simulink model "model_sim_CHBjt7"  (R2023b)
settings: Solver=ode3  StartTime=0.0  StopTime=5  FixedStep=01e-6  RelTol=1e-3
InitFcn:
  | sysinit
StopFcn:
  | code_CHBJT7_stopfcn
values from neighbouring files (symbols this model uses):
  C = 0.0234    [sysinit.m]
  f = 50    [sysinit.m]
  f_switch = 250    [sysinit.m]
  fn = 50    [sysinit.m]
  L = 0.002    [sysinit.m]
  L_1 = eps    [simout_chb_par.m]    (also in simout_chbjt_par.m; sysinit.m)
  L_ori = 0.02    [sysinit.m]
  L_sec = 0.06    [sysinit.m]
  m = 0.95    [sysinit.m]
  P0 = 8e6    (= 8000000)    [sysinit.m]
  R = 1.5    [sysinit.m]
  Source_Amp = 10000    [sysinit.m]
  st = 1e-6    (= 1e-06)    [sysinit.m]
  Td = 15e-7    (= 1.5e-06)    [sysinit.m]
  Ts2 = 0.5e-3    (= 0.0005)    [sysinit.m]
  U_dcN = 2500    [sysinit.m]
  Ul_in = 1900    [sysinit.m]
undefined symbols (not defined in the file or in its folder): magnitude
libraries: spsSeriesRLCBranchLib x120, spsDiodeLib x45, spsIGBTLib x36, spsMeanLib x20, spsCurrentMeasurementLib x15, spsThreePhaseVIMeasurementLib x10, spsOnDelayLib x9, spsMultiWindingTransformerLib x9, spsUniversalBridgeLib x9, simulink x5, spsVoltageMeasurementLib x5, spsRMSLib x4
(part 3 of 3)

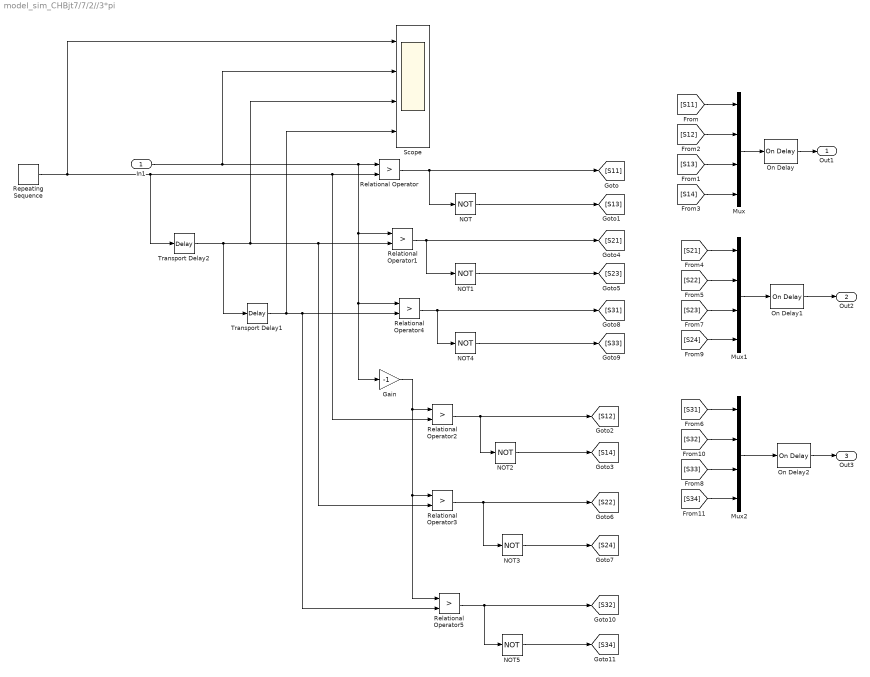
== system model_sim_CHBjt7/7/2//3*pi ==
  In1 : Inport
  Gain : Gain  Gain=-1
  Mux : Mux
  Mux1 : Mux
  Mux2 : Mux
  NOT{,1..5} (6 alike) : Logic  Operator=NOT  AllPortsSameDT=off  OutDataTypeStr=boolean
  On Delay : spsOnDelayLib/On Delay  DelayType=On delay  delay=ttd  ic=0  Ts=0
  On Delay1 : spsOnDelayLib/On Delay  DelayType=On delay  delay=ttd  ic=0  Ts=0
  On Delay2 : spsOnDelayLib/On Delay  DelayType=On delay  delay=ttd  ic=0  Ts=0
  Relational Operator{,1..5} (6 alike) : RelationalOperator  Operator=>  OutDataTypeStr=boolean  RndMeth=Simplest  InputSameDT=off
  Repeating Sequence : simulink/Sources/Repeating Sequence  rep_seq_t=[0 0.5 1]/f_car  rep_seq_y=[-1 1 -1]*1000
  Scope : Scope  NumInputPorts=4
  Transport Delay1 : TransportDelay  DelayTime=tt/f_car  BufferSize=3072
  Transport Delay2 : TransportDelay  DelayTime=tt/f_car  BufferSize=3072
  Out1 : Outport
  Out2 : Outport  Port=2
  Out3 : Outport  Port=3
  wires:
  NOT/1 -> [S13]
  Transport Delay2/1 -> Scope/3, Relational Operator3/2, Relational Operator1/2, Transport Delay1/1
  [S14] -> Mux/4
  [S23] -> Mux1/3
  [S12] -> Mux/2
  In1/1 -> Scope/2, Relational Operator4/1, Gain/1, Relational Operator1/1, Relational Operator/1
  [S34] -> Mux2/4
  [S32] -> Mux2/2
  Mux2/1 -> On Delay2/1
  Relational Operator5/1 -> [S32], NOT5/1
  NOT2/1 -> [S14]
  [S21] -> Mux1/1
  NOT4/1 -> [S33]
  Relational Operator1/1 -> NOT1/1, [S21]
  [S22] -> Mux1/2
  [S33] -> Mux2/3
  NOT3/1 -> [S24]
  Mux/1 -> On Delay/1
  [S24] -> Mux1/4
  Relational Operator4/1 -> [S31], NOT4/1
  Gain/1 -> Relational Operator5/1, Relational Operator3/1, Relational Operator2/1
  [S13] -> Mux/3
  Relational Operator2/1 -> NOT2/1, [S12]
  [S31] -> Mux2/1
  [S11] -> Mux/1
  NOT5/1 -> [S34]
  Relational Operator/1 -> NOT/1, [S11]
  NOT1/1 -> [S23]
  Mux1/1 -> On Delay1/1
  Relational Operator3/1 -> NOT3/1, [S22]
  On Delay/1 -> Out1/1
  On Delay1/1 -> Out2/1
  On Delay2/1 -> Out3/1
  Transport Delay1/1 -> Scope/4, Relational Operator5/2, Relational Operator4/2
  Repeating Sequence/1 -> Scope/1, Transport Delay2/1, Relational Operator2/2, Relational Operator/2

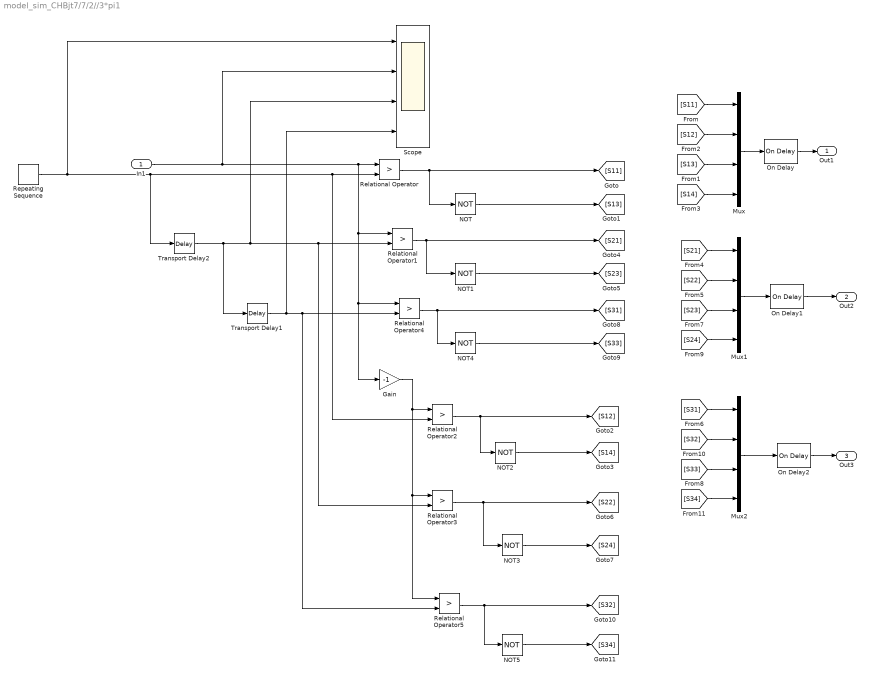
== system model_sim_CHBjt7/7/2//3*pi1 ==
  In1 : Inport
  Gain : Gain  Gain=-1
  Mux : Mux
  Mux1 : Mux
  Mux2 : Mux
  NOT{,1..5} (6 alike) : Logic  Operator=NOT  AllPortsSameDT=off  OutDataTypeStr=boolean
  On Delay : spsOnDelayLib/On Delay  DelayType=On delay  delay=ttd  ic=0  Ts=0
  On Delay1 : spsOnDelayLib/On Delay  DelayType=On delay  delay=ttd  ic=0  Ts=0
  On Delay2 : spsOnDelayLib/On Delay  DelayType=On delay  delay=ttd  ic=0  Ts=0
  Relational Operator{,1..5} (6 alike) : RelationalOperator  Operator=>  OutDataTypeStr=boolean  RndMeth=Simplest  InputSameDT=off
  Repeating Sequence : simulink/Sources/Repeating Sequence  rep_seq_t=[0 0.5 1]/f_car  rep_seq_y=[-1 1 -1]*1000
  Scope : Scope  NumInputPorts=4
  Transport Delay1 : TransportDelay  DelayTime=tt/f_car  BufferSize=3072
  Transport Delay2 : TransportDelay  DelayTime=tt/f_car  BufferSize=3072
  Out1 : Outport
  Out2 : Outport  Port=2
  Out3 : Outport  Port=3
  wires:
  NOT/1 -> [S13]
  Transport Delay2/1 -> Scope/3, Relational Operator3/2, Relational Operator1/2, Transport Delay1/1
  [S14] -> Mux/4
  [S23] -> Mux1/3
  [S12] -> Mux/2
  In1/1 -> Scope/2, Relational Operator4/1, Gain/1, Relational Operator1/1, Relational Operator/1
  [S34] -> Mux2/4
  [S32] -> Mux2/2
  Mux2/1 -> On Delay2/1
  Relational Operator5/1 -> [S32], NOT5/1
  NOT2/1 -> [S14]
  [S21] -> Mux1/1
  NOT4/1 -> [S33]
  Relational Operator1/1 -> NOT1/1, [S21]
  [S22] -> Mux1/2
  [S33] -> Mux2/3
  NOT3/1 -> [S24]
  Mux/1 -> On Delay/1
  [S24] -> Mux1/4
  Relational Operator4/1 -> [S31], NOT4/1
  Gain/1 -> Relational Operator5/1, Relational Operator3/1, Relational Operator2/1
  [S13] -> Mux/3
  Relational Operator2/1 -> NOT2/1, [S12]
  [S31] -> Mux2/1
  [S11] -> Mux/1
  NOT5/1 -> [S34]
  Relational Operator/1 -> NOT/1, [S11]
  NOT1/1 -> [S23]
  Mux1/1 -> On Delay1/1
  Relational Operator3/1 -> NOT3/1, [S22]
  On Delay/1 -> Out1/1
  On Delay1/1 -> Out2/1
  On Delay2/1 -> Out3/1
  Transport Delay1/1 -> Scope/4, Relational Operator5/2, Relational Operator4/2
  Repeating Sequence/1 -> Scope/1, Transport Delay2/1, Relational Operator2/2, Relational Operator/2

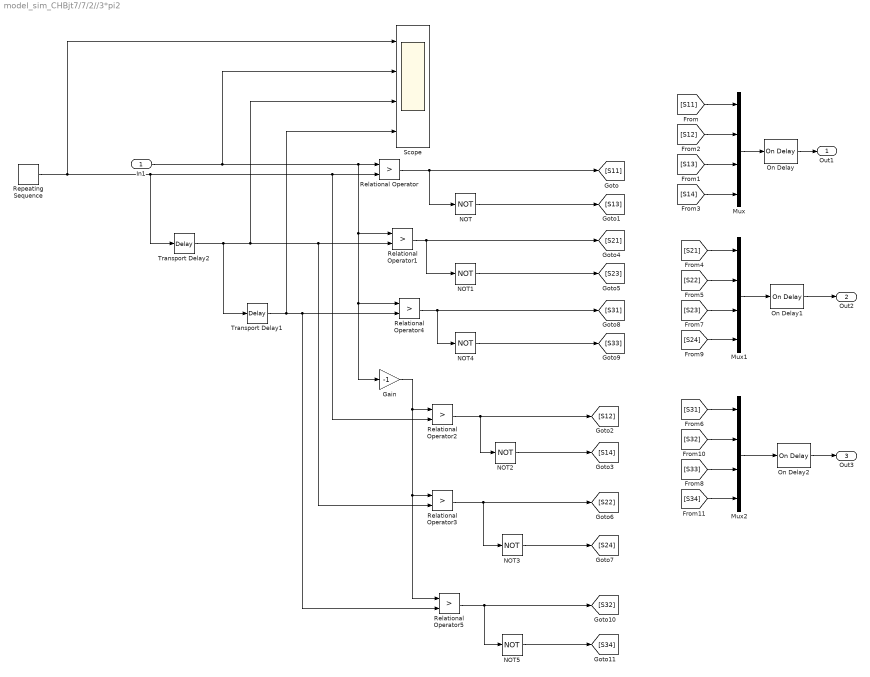
== system model_sim_CHBjt7/7/2//3*pi2 ==
  In1 : Inport
  Gain : Gain  Gain=-1
  Mux : Mux
  Mux1 : Mux
  Mux2 : Mux
  NOT{,1..5} (6 alike) : Logic  Operator=NOT  AllPortsSameDT=off  OutDataTypeStr=boolean
  On Delay : spsOnDelayLib/On Delay  DelayType=On delay  delay=ttd  ic=0  Ts=0
  On Delay1 : spsOnDelayLib/On Delay  DelayType=On delay  delay=ttd  ic=0  Ts=0
  On Delay2 : spsOnDelayLib/On Delay  DelayType=On delay  delay=ttd  ic=0  Ts=0
  Relational Operator{,1..5} (6 alike) : RelationalOperator  Operator=>  OutDataTypeStr=boolean  RndMeth=Simplest  InputSameDT=off
  Repeating Sequence : simulink/Sources/Repeating Sequence  rep_seq_t=[0 0.5 1]/f_car  rep_seq_y=[-1 1 -1]*1000
  Scope : Scope  NumInputPorts=4
  Transport Delay1 : TransportDelay  DelayTime=tt/f_car  BufferSize=3072
  Transport Delay2 : TransportDelay  DelayTime=tt/f_car  BufferSize=3072
  Out1 : Outport
  Out2 : Outport  Port=2
  Out3 : Outport  Port=3
  wires:
  NOT/1 -> [S13]
  Transport Delay2/1 -> Scope/3, Relational Operator3/2, Relational Operator1/2, Transport Delay1/1
  [S14] -> Mux/4
  [S23] -> Mux1/3
  [S12] -> Mux/2
  In1/1 -> Scope/2, Relational Operator4/1, Gain/1, Relational Operator1/1, Relational Operator/1
  [S34] -> Mux2/4
  [S32] -> Mux2/2
  Mux2/1 -> On Delay2/1
  Relational Operator5/1 -> [S32], NOT5/1
  NOT2/1 -> [S14]
  [S21] -> Mux1/1
  NOT4/1 -> [S33]
  Relational Operator1/1 -> NOT1/1, [S21]
  [S22] -> Mux1/2
  [S33] -> Mux2/3
  NOT3/1 -> [S24]
  Mux/1 -> On Delay/1
  [S24] -> Mux1/4
  Relational Operator4/1 -> [S31], NOT4/1
  Gain/1 -> Relational Operator5/1, Relational Operator3/1, Relational Operator2/1
  [S13] -> Mux/3
  Relational Operator2/1 -> NOT2/1, [S12]
  [S31] -> Mux2/1
  [S11] -> Mux/1
  NOT5/1 -> [S34]
  Relational Operator/1 -> NOT/1, [S11]
  NOT1/1 -> [S23]
  Mux1/1 -> On Delay1/1
  Relational Operator3/1 -> NOT3/1, [S22]
  On Delay/1 -> Out1/1
  On Delay1/1 -> Out2/1
  On Delay2/1 -> Out3/1
  Transport Delay1/1 -> Scope/4, Relational Operator5/2, Relational Operator4/2
  Repeating Sequence/1 -> Scope/1, Transport Delay2/1, Relational Operator2/2, Relational Operator/2

== system model_sim_CHBjt7/7/Subsystem ==
  In1 : Inport
  In2 : Inport  Port=2
  In3 : Inport  Port=3
  Add{1..3,9} (4 alike) : Sum
  Gain : Gain  Gain=-0.5
  Max : MinMax  Function=max  Inputs=3
  Max1 : MinMax  Inputs=3
  Out1 : Outport
  Out2 : Outport  Port=2
  Out3 : Outport  Port=3
  wires:
  In2/1 -> Add3/2, Max1/2, Max/2
  In3/1 -> Add9/2, Max1/3, Max/3
  In1/1 -> Max1/1, Add2/2, Max/1
  Gain/1 -> Add9/1, Add3/1, Add2/1
  Max/1 -> Add1/1
  Max1/1 -> Add1/2
  Add1/1 -> Gain/1
  Add9/1 -> Out3/1
  Add2/1 -> Out1/1
  Add3/1 -> Out2/1

== system model_sim_CHBjt7/JUNCTION TEMP/Subsystem14 ==
  In1 : Inport
  In2 : Inport  Port=2
  Add : Sum
  Constant : Constant  Value=0
  Constant1 : Constant  Value=0
  Gain1 : Gain  Gain=0.39e-3
  Gain2 : Gain  Gain=1.39
  Gain3 : Gain
  Logical Operator : Logic  AllPortsSameDT=off  OutDataTypeStr=boolean
  Math Function : Math  Operator=magnitude^2  SignedPower=on
  Relational Operator : RelationalOperator  Operator=>  OutDataTypeStr=boolean  RndMeth=Simplest  InputSameDT=off
  Switch13 : Switch  Criteria=u2 > Threshold  SaturateOnIntegerOverflow=off  InputSameDT=off
  t1_temper{1..4} (4 alike) : Scope
  Out1 : Outport  VectorParamsAs1DForOutWhenUnconnected=off
  wires:
  Add/1 -> t1_temper4/1, Switch13/1
  Gain2/1 -> Add/2
  Math Function/1 -> Gain1/1
  In1/1 -> t1_temper3/1, Relational Operator/1, Gain3/1
  Gain1/1 -> Add/1
  Gain3/1 -> Gain2/1, Math Function/1
  Constant/1 -> Relational Operator/2
  Relational Operator/1 -> Logical Operator/1
  In2/1 -> t1_temper1/1, Logical Operator/2
  Logical Operator/1 -> t1_temper2/1, Switch13/2
  Switch13/1 -> Out1/1
  Constant1/1 -> Switch13/3

== system model_sim_CHBjt7/JUNCTION TEMP/Subsystem15 ==
  In1 : Inport
  In2 : Inport  Port=2
  Add1 : Sum  Inputs=5
  Add2 : Sum  Inputs=+++
  Add3 : Sum
  Constant1 : Constant  Value=40
  Discrete Filter1 : DiscreteFilter  Numerator=[Ts2/0.3]  Denominator=[1 (Ts2/0.3)-1]  SampleTime=Ts2
  Discrete Filter5 : DiscreteFilter  Numerator=[Ts2/605e-3]  Denominator=[1 (Ts2/605e-3)-1]  SampleTime=Ts2
  Discrete Filter6 : DiscreteFilter  Numerator=[Ts2/101e-3]  Denominator=[1 (Ts2/101e-3)-1]  SampleTime=Ts2
  Discrete Filter7 : DiscreteFilter  Numerator=[Ts2/5.2e-3]  Denominator=[1 (Ts2/5.2e-3)-1]  SampleTime=Ts2
  Discrete Filter8 : DiscreteFilter  Numerator=[Ts2/0.6e-3]  Denominator=[1 (Ts2/0.6e-3)-1]  SampleTime=Ts2
  Discrete Filter9 : DiscreteFilter  Numerator=[Ts2/0.5]  Denominator=[1 (Ts2/0.5)-1]  SampleTime=Ts2
  Gain1 : Gain  Gain=2.4e-3
  Gain5 : Gain  Gain=3.45e-3
  Gain6 : Gain  Gain=2.26e-3
  Gain7 : Gain  Gain=0.97e-3
  Gain8 : Gain  Gain=0.1e-3
  Gain9 : Gain  Gain=7.5e-3
  Out1 : Outport  VectorParamsAs1DForOutWhenUnconnected=off
  wires:
  In1/1 -> Add3/1
  In2/1 -> Add3/2
  Gain6/1 -> Discrete Filter6/1
  Gain9/1 -> Discrete Filter9/1
  Discrete Filter9/1 -> Add2/1
  Gain5/1 -> Discrete Filter5/1
  Discrete Filter6/1 -> Add1/2
  Gain7/1 -> Discrete Filter7/1
  Constant1/1 -> Add2/3
  Discrete Filter7/1 -> Add1/3
  Discrete Filter8/1 -> Add1/4
  Discrete Filter5/1 -> Add1/1
  Gain8/1 -> Discrete Filter8/1
  Add1/1 -> Add2/2
  Add2/1 -> Out1/1
  Discrete Filter1/1 -> Add1/5
  Gain1/1 -> Discrete Filter1/1
  Add3/1 -> Gain5/1, Gain9/1, Gain6/1, Gain7/1, Gain1/1, Gain8/1

== system model_sim_CHBjt7/JUNCTION TEMP/Subsystem16 ==
  In1 : Inport
  In2 : Inport  Port=2
  Abs1 : Abs  SaturateOnIntegerOverflow=off
  Add : Sum
  Constant1 : Constant  Value=0
  Constant2 : Constant  Value=0
  Gain1 : Gain  Gain=21.5/4000*U_dcN/2800
  Gain2 : Gain  Gain=3/4000*U_dcN/2800
  Gain3 : Gain  Gain=1/Ts2
  Gain4 : Gain
  Logical Operator : Logic  AllPortsSameDT=off  OutDataTypeStr=boolean
  Logical Operator1 : Logic  Operator=NOT  AllPortsSameDT=off  OutDataTypeStr=boolean
  Logical Operator2 : Logic  Operator=NOT  AllPortsSameDT=off  OutDataTypeStr=boolean
  Logical Operator3 : Logic  AllPortsSameDT=off  OutDataTypeStr=boolean
  Logical Operator4 : Logic  AllPortsSameDT=off  OutDataTypeStr=boolean
  Logical Operator5 : Logic  Operator=NOT  AllPortsSameDT=off  OutDataTypeStr=boolean
  Pulse Generator : DiscretePulseGenerator  PulseType=Time based  Period=Ts2  PulseWidth=5
  Scope1 : Scope  NumInputPorts=3
  Scope7 : Scope  NumInputPorts=2
  Switch{1..4} (4 alike) : Switch  Criteria=u2 > Threshold  SaturateOnIntegerOverflow=off  InputSameDT=off
  Unit Delay{,1..3} (4 alike) : UnitDelay  SampleTime=1e-6  HasFrameUpgradeWarning=on
  Out1 : Outport  VectorParamsAs1DForOutWhenUnconnected=off
  wires:
  In2/1 -> Logical Operator2/1, Logical Operator/1, Unit Delay/1
  Logical Operator/1 -> Switch1/2
  Abs1/1 -> Add/1
  Switch2/1 -> Gain1/1
  Switch1/1 -> Scope1/1, Abs1/1
  Unit Delay/1 -> Logical Operator3/1, Logical Operator1/1
  Logical Operator1/1 -> Logical Operator/2
  Logical Operator2/1 -> Logical Operator3/2
  Logical Operator3/1 -> Switch2/2
  Constant2/1 -> Switch2/3
  Gain2/1 -> Switch1/1
  Gain1/1 -> Switch1/3
  Switch3/1 -> Add/2
  Constant1/1 -> Switch3/1
  Pulse Generator/1 -> Unit Delay3/1, Logical Operator4/1
  Switch4/1 -> Scope7/2, Unit Delay2/1, Gain3/1
  Unit Delay2/1 -> Switch4/3
  Unit Delay3/1 -> Logical Operator5/1
  Logical Operator5/1 -> Logical Operator4/2
  Logical Operator4/1 -> Scope1/3, Switch4/2, Switch3/2
  Unit Delay1/1 -> Scope7/1, Switch3/3, Switch4/1
  Gain3/1 -> Out1/1
  In1/1 -> Gain4/1
  Add/1 -> Scope1/2, Unit Delay1/1
  Gain4/1 -> Switch2/1, Gain2/1

== system model_sim_CHBjt7/JUNCTION TEMP/Subsystem17 ==
  In1 : Inport
  In2 : Inport  Port=2
  Add : Sum
  Constant : Constant  Value=0
  Constant1 : Constant  Value=0
  Gain1 : Gain  Gain=0.39e-3
  Gain2 : Gain  Gain=1.39
  Gain3 : Gain
  Logical Operator : Logic  AllPortsSameDT=off  OutDataTypeStr=boolean
  Math Function : Math  Operator=magnitude^2  SignedPower=on
  Relational Operator : RelationalOperator  Operator=>  OutDataTypeStr=boolean  RndMeth=Simplest  InputSameDT=off
  Switch13 : Switch  Criteria=u2 > Threshold  SaturateOnIntegerOverflow=off  InputSameDT=off
  t1_temper{1..4} (4 alike) : Scope
  Out1 : Outport  VectorParamsAs1DForOutWhenUnconnected=off
  wires:
  Add/1 -> t1_temper4/1, Switch13/1
  Gain2/1 -> Add/2
  Math Function/1 -> Gain1/1
  In1/1 -> t1_temper3/1, Relational Operator/1, Gain3/1
  Gain1/1 -> Add/1
  Gain3/1 -> Gain2/1, Math Function/1
  Constant/1 -> Relational Operator/2
  Relational Operator/1 -> Logical Operator/1
  In2/1 -> t1_temper1/1, Logical Operator/2
  Logical Operator/1 -> t1_temper2/1, Switch13/2
  Switch13/1 -> Out1/1
  Constant1/1 -> Switch13/3

== system model_sim_CHBjt7/JUNCTION TEMP/Subsystem18 ==
  In1 : Inport
  In2 : Inport  Port=2
  Add1 : Sum  Inputs=5
  Add2 : Sum  Inputs=+++
  Add3 : Sum
  Constant1 : Constant  Value=40
  Discrete Filter1 : DiscreteFilter  Numerator=[Ts2/0.3]  Denominator=[1 (Ts2/0.3)-1]  SampleTime=Ts2
  Discrete Filter5 : DiscreteFilter  Numerator=[Ts2/605e-3]  Denominator=[1 (Ts2/605e-3)-1]  SampleTime=Ts2
  Discrete Filter6 : DiscreteFilter  Numerator=[Ts2/101e-3]  Denominator=[1 (Ts2/101e-3)-1]  SampleTime=Ts2
  Discrete Filter7 : DiscreteFilter  Numerator=[Ts2/5.2e-3]  Denominator=[1 (Ts2/5.2e-3)-1]  SampleTime=Ts2
  Discrete Filter8 : DiscreteFilter  Numerator=[Ts2/0.6e-3]  Denominator=[1 (Ts2/0.6e-3)-1]  SampleTime=Ts2
  Discrete Filter9 : DiscreteFilter  Numerator=[Ts2/0.5]  Denominator=[1 (Ts2/0.5)-1]  SampleTime=Ts2
  Gain1 : Gain  Gain=2.4e-3
  Gain5 : Gain  Gain=3.45e-3
  Gain6 : Gain  Gain=2.26e-3
  Gain7 : Gain  Gain=0.97e-3
  Gain8 : Gain  Gain=0.1e-3
  Gain9 : Gain  Gain=7.5e-3
  Out1 : Outport  VectorParamsAs1DForOutWhenUnconnected=off
  wires:
  In1/1 -> Add3/1
  In2/1 -> Add3/2
  Gain6/1 -> Discrete Filter6/1
  Gain9/1 -> Discrete Filter9/1
  Discrete Filter9/1 -> Add2/1
  Gain5/1 -> Discrete Filter5/1
  Discrete Filter6/1 -> Add1/2
  Gain7/1 -> Discrete Filter7/1
  Constant1/1 -> Add2/3
  Discrete Filter7/1 -> Add1/3
  Discrete Filter8/1 -> Add1/4
  Discrete Filter5/1 -> Add1/1
  Gain8/1 -> Discrete Filter8/1
  Add1/1 -> Add2/2
  Add2/1 -> Out1/1
  Discrete Filter1/1 -> Add1/5
  Gain1/1 -> Discrete Filter1/1
  Add3/1 -> Gain5/1, Gain9/1, Gain6/1, Gain7/1, Gain1/1, Gain8/1

== system model_sim_CHBjt7/JUNCTION TEMP/Subsystem48 ==
  In1 : Inport
  In2 : Inport  Port=2
  Abs1 : Abs  SaturateOnIntegerOverflow=off
  Add : Sum
  Constant1 : Constant  Value=0
  Constant2 : Constant  Value=0
  Fcn2 : Fcn  Expr=-2.8E-7*u*u+0.00278*u+3.056
  Gain1 : Gain  Gain=U_dcN/2800*11.5/13
  Gain2 : Gain  Gain=4.1/500
  Gain3 : Gain  Gain=1/Ts2
  Gain4 : Gain
  Logical Operator2 : Logic  Operator=NOT  AllPortsSameDT=off  OutDataTypeStr=boolean
  Logical Operator3 : Logic  AllPortsSameDT=off  OutDataTypeStr=boolean
  Logical Operator4 : Logic  AllPortsSameDT=off  OutDataTypeStr=boolean
  Logical Operator5 : Logic  Operator=NOT  AllPortsSameDT=off  OutDataTypeStr=boolean
  Pulse Generator : DiscretePulseGenerator  PulseType=Time based  Period=Ts2  PulseWidth=5
  Saturation : Saturate  UpperLimit=5500  LowerLimit=0
  Saturation1 : Saturate  UpperLimit=100  LowerLimit=0
  Scope1 : Scope  NumInputPorts=3
  Scope7 : Scope  NumInputPorts=2
  Switch1 : Switch  Criteria=u2 > Threshold  Threshold=500  SaturateOnIntegerOverflow=off  InputSameDT=off
  Switch2 : Switch  Criteria=u2 > Threshold  SaturateOnIntegerOverflow=off  InputSameDT=off
  Switch3 : Switch  Criteria=u2 > Threshold  SaturateOnIntegerOverflow=off  InputSameDT=off
  Switch4 : Switch  Criteria=u2 > Threshold  SaturateOnIntegerOverflow=off  InputSameDT=off
  Unit Delay{,1..3} (4 alike) : UnitDelay  SampleTime=1e-6  HasFrameUpgradeWarning=on
  Out1 : Outport  VectorParamsAs1DForOutWhenUnconnected=off
  wires:
  Abs1/1 -> Add/1
  Switch2/1 -> Gain1/1
  Gain1/1 -> Abs1/1, Scope1/1
  In2/1 -> Logical Operator3/1, Unit Delay/1
  Logical Operator2/1 -> Logical Operator3/2
  Logical Operator3/1 -> Switch2/2
  Constant2/1 -> Switch2/3
  Switch3/1 -> Add/2
  Constant1/1 -> Switch3/1
  Pulse Generator/1 -> Unit Delay3/1, Logical Operator4/1
  Switch4/1 -> Scope7/2, Unit Delay2/1, Gain3/1
  Unit Delay2/1 -> Switch4/3
  Unit Delay3/1 -> Logical Operator5/1
  Logical Operator5/1 -> Logical Operator4/2
  Logical Operator4/1 -> Scope1/3, Switch4/2, Switch3/2
  Unit Delay1/1 -> Scope7/1, Switch3/3, Switch4/1
  Gain3/1 -> Out1/1
  In1/1 -> Gain4/1
  Add/1 -> Scope1/2, Unit Delay1/1
  Unit Delay/1 -> Logical Operator2/1
  Fcn2/1 -> Switch1/1
  Gain4/1 -> Saturation/1
  Saturation/1 -> Fcn2/1, Switch1/2, Gain2/1
  Saturation1/1 -> Switch2/1
  Gain2/1 -> Switch1/3
  Switch1/1 -> Saturation1/1

== system model_sim_CHBjt7/JUNCTION TEMP/Subsystem49 ==
  In1 : Inport
  In2 : Inport  Port=2
  Add3 : Sum
  Add4 : Sum  Inputs=5
  Add5 : Sum  Inputs=+++
  Constant : Constant  Value=40
  Discrete Filter1 : DiscreteFilter  Numerator=[Ts2/5e-3]  Denominator=[1 (Ts2/5e-3)-1]  SampleTime=Ts2
  Discrete Filter2 : DiscreteFilter  Numerator=[Ts2/100e-3]  Denominator=[1 (Ts2/100e-3)-1]  SampleTime=Ts2
  Discrete Filter3 : DiscreteFilter  Numerator=[Ts2/800e-3]  Denominator=[1 (Ts2/800e-3)-1]  SampleTime=Ts2
  Discrete Filter4 : DiscreteFilter  Numerator=[Ts2/0.5]  Denominator=[1 (Ts2/0.5)-1]  SampleTime=Ts2
  Discrete Filter5 : DiscreteFilter  Numerator=[Ts2/300e-3]  Denominator=[1 (Ts2/300e-3)-1]  SampleTime=Ts2
  Gain1 : Gain  Gain=0.44e-3
  Gain2 : Gain  Gain=2.255e-3
  Gain3 : Gain  Gain=2.915e-3
  Gain4 : Gain  Gain=7.5e-3
  Gain5 : Gain  Gain=2.2e-3
  t1_temper : Scope
  t1_temper1 : Scope
  Out1 : Outport  VectorParamsAs1DForOutWhenUnconnected=off
  wires:
  In1/1 -> Add3/1
  Gain2/1 -> Discrete Filter2/1
  Discrete Filter2/1 -> Add4/3
  Discrete Filter3/1 -> Add4/4
  Add4/1 -> Add5/2
  Gain3/1 -> Discrete Filter3/1
  Add3/1 -> Gain5/1, t1_temper/1, Gain3/1, Gain4/1, Gain1/1, Gain2/1
  In2/1 -> Add3/2
  Constant/1 -> Add5/3
  Gain1/1 -> Discrete Filter1/1
  Gain4/1 -> Discrete Filter4/1
  Add5/1 -> Out1/1
  Discrete Filter1/1 -> Add4/2
  Discrete Filter4/1 -> t1_temper1/1, Add5/1
  Gain5/1 -> Discrete Filter5/1
  Discrete Filter5/1 -> Add4/5

== system model_sim_CHBjt7/JUNCTION TEMP/Subsystem5 ==
  In1 : Inport
  In2 : Inport  Port=2
  Abs1 : Abs  SaturateOnIntegerOverflow=off
  Add : Sum
  Constant1 : Constant  Value=0
  Constant2 : Constant  Value=0
  Fcn2 : Fcn  Expr=-2.8E-7*u*u+0.00278*u+3.056
  Gain1 : Gain  Gain=U_dcN/2800*11.5/13
  Gain2 : Gain  Gain=4.1/500
  Gain3 : Gain  Gain=1/Ts2
  Gain4 : Gain
  Logical Operator2 : Logic  Operator=NOT  AllPortsSameDT=off  OutDataTypeStr=boolean
  Logical Operator3 : Logic  AllPortsSameDT=off  OutDataTypeStr=boolean
  Logical Operator4 : Logic  AllPortsSameDT=off  OutDataTypeStr=boolean
  Logical Operator5 : Logic  Operator=NOT  AllPortsSameDT=off  OutDataTypeStr=boolean
  Pulse Generator : DiscretePulseGenerator  PulseType=Time based  Period=Ts2  PulseWidth=5
  Saturation : Saturate  UpperLimit=5500  LowerLimit=0
  Saturation1 : Saturate  UpperLimit=100  LowerLimit=0
  Scope1 : Scope  NumInputPorts=3
  Scope7 : Scope  NumInputPorts=2
  Switch1 : Switch  Criteria=u2 > Threshold  Threshold=500  SaturateOnIntegerOverflow=off  InputSameDT=off
  Switch2 : Switch  Criteria=u2 > Threshold  SaturateOnIntegerOverflow=off  InputSameDT=off
  Switch3 : Switch  Criteria=u2 > Threshold  SaturateOnIntegerOverflow=off  InputSameDT=off
  Switch4 : Switch  Criteria=u2 > Threshold  SaturateOnIntegerOverflow=off  InputSameDT=off
  Unit Delay{,1..3} (4 alike) : UnitDelay  SampleTime=1e-6  HasFrameUpgradeWarning=on
  Out1 : Outport  VectorParamsAs1DForOutWhenUnconnected=off
  wires:
  Switch1/1 -> Saturation1/1
  Gain2/1 -> Switch1/3
  Saturation1/1 -> Switch2/1
  Saturation/1 -> Gain2/1, Switch1/2, Fcn2/1
  Gain4/1 -> Saturation/1
  Fcn2/1 -> Switch1/1
  Unit Delay/1 -> Logical Operator2/1
  Add/1 -> Unit Delay1/1, Scope1/2
  In1/1 -> Gain4/1
  Gain3/1 -> Out1/1
  Unit Delay1/1 -> Switch4/1, Switch3/3, Scope7/1
  Logical Operator4/1 -> Switch3/2, Switch4/2, Scope1/3
  Logical Operator5/1 -> Logical Operator4/2
  Unit Delay3/1 -> Logical Operator5/1
  Unit Delay2/1 -> Switch4/3
  Switch4/1 -> Gain3/1, Unit Delay2/1, Scope7/2
  Pulse Generator/1 -> Logical Operator4/1, Unit Delay3/1
  Constant1/1 -> Switch3/1
  Switch3/1 -> Add/2
  Constant2/1 -> Switch2/3
  Logical Operator3/1 -> Switch2/2
  Logical Operator2/1 -> Logical Operator3/2
  In2/1 -> Unit Delay/1, Logical Operator3/1
  Gain1/1 -> Scope1/1, Abs1/1
  Switch2/1 -> Gain1/1
  Abs1/1 -> Add/1

== system model_sim_CHBjt7/JUNCTION TEMP/Subsystem6 ==
  In1 : Inport
  In2 : Inport  Port=2
  Add3 : Sum
  Add4 : Sum  Inputs=5
  Add5 : Sum  Inputs=+++
  Constant : Constant  Value=40
  Discrete Filter1 : DiscreteFilter  Numerator=[Ts2/5e-3]  Denominator=[1 (Ts2/5e-3)-1]  SampleTime=Ts2
  Discrete Filter2 : DiscreteFilter  Numerator=[Ts2/100e-3]  Denominator=[1 (Ts2/100e-3)-1]  SampleTime=Ts2
  Discrete Filter3 : DiscreteFilter  Numerator=[Ts2/800e-3]  Denominator=[1 (Ts2/800e-3)-1]  SampleTime=Ts2
  Discrete Filter4 : DiscreteFilter  Numerator=[Ts2/0.5]  Denominator=[1 (Ts2/0.5)-1]  SampleTime=Ts2
  Discrete Filter5 : DiscreteFilter  Numerator=[Ts2/300e-3]  Denominator=[1 (Ts2/300e-3)-1]  SampleTime=Ts2
  Gain1 : Gain  Gain=0.44e-3
  Gain2 : Gain  Gain=2.255e-3
  Gain3 : Gain  Gain=2.915e-3
  Gain4 : Gain  Gain=7.5e-3
  Gain5 : Gain  Gain=2.2e-3
  t1_temper : Scope
  t1_temper1 : Scope
  Out1 : Outport  VectorParamsAs1DForOutWhenUnconnected=off
  wires:
  Discrete Filter5/1 -> Add4/5
  Gain5/1 -> Discrete Filter5/1
  Discrete Filter4/1 -> Add5/1, t1_temper1/1
  Discrete Filter1/1 -> Add4/2
  Add5/1 -> Out1/1
  Gain4/1 -> Discrete Filter4/1
  Gain1/1 -> Discrete Filter1/1
  Constant/1 -> Add5/3
  In2/1 -> Add3/2
  Add3/1 -> Gain2/1, Gain1/1, Gain4/1, Gain3/1, t1_temper/1, Gain5/1
  Gain3/1 -> Discrete Filter3/1
  Add4/1 -> Add5/2
  Discrete Filter3/1 -> Add4/4
  Discrete Filter2/1 -> Add4/3
  Gain2/1 -> Discrete Filter2/1
  In1/1 -> Add3/1

== system model_sim_CHBjt7/JUNCTION TEMP/Subsystem9 ==
  In1 : Inport
  In2 : Inport  Port=2
  Abs1 : Abs  SaturateOnIntegerOverflow=off
  Add : Sum
  Constant1 : Constant  Value=0
  Constant2 : Constant  Value=0
  Gain1 : Gain  Gain=21.5/4000*U_dcN/2800
  Gain2 : Gain  Gain=3/4000*U_dcN/2800
  Gain3 : Gain  Gain=1/Ts2
  Gain4 : Gain
  Logical Operator : Logic  AllPortsSameDT=off  OutDataTypeStr=boolean
  Logical Operator1 : Logic  Operator=NOT  AllPortsSameDT=off  OutDataTypeStr=boolean
  Logical Operator2 : Logic  Operator=NOT  AllPortsSameDT=off  OutDataTypeStr=boolean
  Logical Operator3 : Logic  AllPortsSameDT=off  OutDataTypeStr=boolean
  Logical Operator4 : Logic  AllPortsSameDT=off  OutDataTypeStr=boolean
  Logical Operator5 : Logic  Operator=NOT  AllPortsSameDT=off  OutDataTypeStr=boolean
  Pulse Generator : DiscretePulseGenerator  PulseType=Time based  Period=Ts2  PulseWidth=5
  Scope1 : Scope  NumInputPorts=3
  Scope7 : Scope  NumInputPorts=2
  Switch{1..4} (4 alike) : Switch  Criteria=u2 > Threshold  SaturateOnIntegerOverflow=off  InputSameDT=off
  Unit Delay{,1..3} (4 alike) : UnitDelay  SampleTime=1e-6  HasFrameUpgradeWarning=on
  Out1 : Outport  VectorParamsAs1DForOutWhenUnconnected=off
  wires:
  In2/1 -> Logical Operator2/1, Logical Operator/1, Unit Delay/1
  Logical Operator/1 -> Switch1/2
  Abs1/1 -> Add/1
  Switch2/1 -> Gain1/1
  Switch1/1 -> Scope1/1, Abs1/1
  Unit Delay/1 -> Logical Operator3/1, Logical Operator1/1
  Logical Operator1/1 -> Logical Operator/2
  Logical Operator2/1 -> Logical Operator3/2
  Logical Operator3/1 -> Switch2/2
  Constant2/1 -> Switch2/3
  Gain2/1 -> Switch1/1
  Gain1/1 -> Switch1/3
  Switch3/1 -> Add/2
  Constant1/1 -> Switch3/1
  Pulse Generator/1 -> Unit Delay3/1, Logical Operator4/1
  Switch4/1 -> Scope7/2, Unit Delay2/1, Gain3/1
  Unit Delay2/1 -> Switch4/3
  Unit Delay3/1 -> Logical Operator5/1
  Logical Operator5/1 -> Logical Operator4/2
  Logical Operator4/1 -> Scope1/3, Switch4/2, Switch3/2
  Unit Delay1/1 -> Scope7/1, Switch3/3, Switch4/1
  Gain3/1 -> Out1/1
  In1/1 -> Gain4/1
  Add/1 -> Scope1/2, Unit Delay1/1
  Gain4/1 -> Switch2/1, Gain2/1
